simulink model "pendulum_simple_model"  (R2025b)
settings: Solver=FixedStepAuto  StartTime=0.0  StopTime=SIM_TIME  FixedStep=STEP_SIZE  RelTol=1e-3
values from neighbouring files (symbols this model uses):
  i0 = 0    [pendulum_sim.m]
  K_lqr = zeros(1,7)    [pendulum_sim.m]
  STEP_CTRL = 1e-3    (= 0.001)    [params.m]
  theta0 = pi - deg2rad(3)    [pendulum_sim.m]
  theta_dot0 = 0    [pendulum_sim.m]
  x0 = 0    [pendulum_sim.m]
  x_dot0 = 0    [pendulum_sim.m]
settings Model: Creator=farfar  LastModifiedBy=farfar

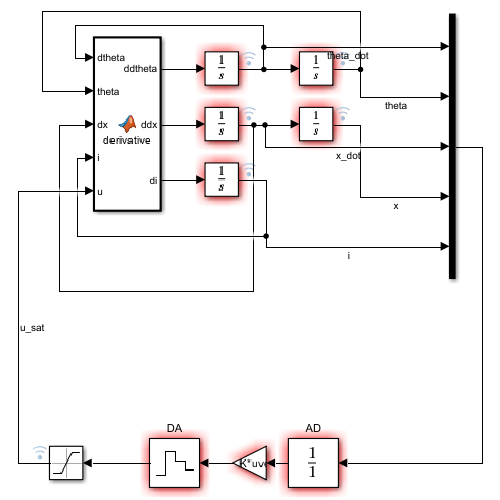
[thumbnail: Simulink's stored preview of the top-level diagram]
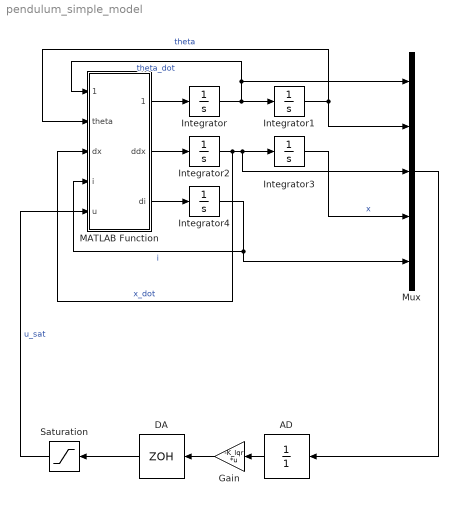
== system pendulum_simple_model ==
  AD : DiscreteTransferFcn  Denominator=[1]  SampleTime=STEP_CTRL
  DA : ZeroOrderHold  SampleTime=STEP_CTRL
  Gain : Gain  Gain=-K_lqr  Multiplication=Matrix(K*u) (u vector)
  Integrator : Integrator  InitialCondition=theta_dot0  ContinuousStateAttributes='dtheta'
  Integrator1 : Integrator  InitialCondition=theta0  ContinuousStateAttributes='theta'
  Integrator2 : Integrator  InitialCondition=x_dot0  ContinuousStateAttributes='dx'
  Integrator3 : Integrator  InitialCondition=x0  ContinuousStateAttributes='x'
  Integrator4 : Integrator  InitialCondition=i0  ContinuousStateAttributes='i'
  MATLAB Function : MATLAB Function  TreatAsAtomicUnit=on
  Mux : Mux  Inputs=5
  Saturation : Saturate  UpperLimit=12  LowerLimit=-12
  wires:
  MATLAB Function/1(ddtheta) -> Integrator/1
  MATLAB Function/2(ddx) -> Integrator2/1
  MATLAB Function/3(di) -> Integrator4/1
  Integrator4/1 -> Mux/5, MATLAB Function/4(i)  "i"
  Integrator1/1 -> Mux/2, MATLAB Function/2(theta)  "theta"
  Integrator/1 -> MATLAB Function/1(dtheta), Mux/1, Integrator1/1  "theta_dot"
  Integrator2/1 -> MATLAB Function/3(dx), Mux/3, Integrator3/1  "x_dot"
  Integrator3/1 -> Mux/4  "x"
  Gain/1 -> DA/1
  AD/1 -> Gain/1
  DA/1 -> Saturation/1
  Mux/1 -> AD/1
  Saturation/1 -> MATLAB Function/5(u)  "u_sat"

== matlab function pendulum_simple_model/MATLAB Function ==
  data: dtheta input; ddtheta output; ddx output; di output; theta input; dx input; i input; u input
function [ddtheta, ddx, di] = derivative(dtheta, theta, dx, i, u)
R = 2.59;     % Resistance (ohm)
L = 708e-6;   % Inductance (H)
J = 115*1e-7; % Rotor inertia (kg m^3) 
Kt = 79.7e-3; % Torque constant (Nm)
Ke = Kt;      % EMF constant V/(rad/s)
d = 0;        % Viscous friction (Nm/(rad/s))
Mr = 6.5e-3;  % Friction torque (Nm)
N = 1; % Gear ratio

% Misc
r = 0.006366197723676;
g = 9.82;       % Gravitational constant (m/s^2)
% Pendulum + cart
Ltotal = 0.4; % Pendulum length (m)
l = Ltotal/2; % Pendulum half length (m)
M = 54e-3; % Cart mass (kg)
m = 7850*Ltotal*(4e-3)^2*pi; % Pendulum mass (kg)
I = (1/3) * m * l^2; % Pendulum inertia (kgm^2)
b = 0; % friction coefficient trolley [kg/s]
c = 0; % friction coefficient pendulum [kg*m^2/s]
% Belt
k_belt = 1e3; % Belt stiffness (N/m)
Meff = (M+m)+J/r^2;
zeta = 0.7;
c_belt = 2*zeta*sqrt(Meff*k_belt); % Belt dampening (Ns/m)


    ddtheta = -(J*c*dtheta + M*c*dtheta*r^2 + c*dtheta*m*r^2 + g*l*m^2*r^2*sin(theta) + J*g*l*m*sin(theta) + (dtheta^2*l^2*m^2*r^2*sin(2*theta))/2 - d*dx*l*m*cos(theta) + Kt*i*l*m*r*cos(theta) + M*g*l*m*r^2*sin(theta) - b*dx*l*m*r^2*cos(theta))/(I*J + I*M*r^2 + l^2*m^2*r^2 + J*l^2*m + I*m*r^2 - l^2*m^2*r^2*cos(theta)^2 + M*l^2*m*r^2);
    ddx = (sin(theta)*dtheta^2*l^3*m^2*r^2 + sin(theta)*I*dtheta^2*l*m*r^2 + c*cos(theta)*dtheta*l*m*r^2 + (g*sin(2*theta)*l^2*m^2*r^2)/2 - b*dx*l^2*m*r^2 + Kt*i*l^2*m*r - d*dx*l^2*m - b*dx*I*r^2 + Kt*i*I*r - d*dx*I)/(I*J + I*M*r^2 + l^2*m^2*r^2 + J*l^2*m + I*m*r^2 - l^2*m^2*r^2*cos(theta)^2 + M*l^2*m*r^2);
    di = -(Ke*dx - r*u + R*i*r)/(L*r);
end
